simulink model "righttrajectoryagent"  (Simulink 6.2)
settings: Solver=ode45  SolverMode=SingleTasking  StartTime=0.0  StopTime=10.0  RelTol=1e-3  AbsTol=1e-6
settings Model: Creator=The MathWorks Inc.  LastModifiedBy=suarezjl  ExtModeTrigMode=oneshot  ExtModeArmWhenConnect=off  ExtModeAutoUpdateStatusClock=off
settings DataIOCC: LimitDataPoints=off  SignalLoggingName=logsOut
settings OptimizationCC: BooleanDataType=off  InlineInvariantSignals=on
settings DebuggingCC: CheckExecutionContextPreStartOutputMsg=on  CheckExecutionContextRuntimeOutputMsg=on  IntegerOverflowMsg=none
settings HardwareCC: TargetUnknown=on
settings ModelReferenceCC: UpdateModelReferenceTargets=IfOutOfDate

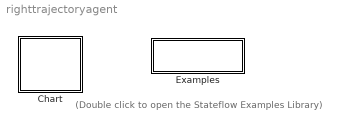
== system righttrajectoryagent ==
  note: (Double click to open the
      | Stateflow Examples Library)
  Chart : Stateflow chart
  Examples : Subsystem
      settings: OpenFcn=sf('Private','sf_examples')
      mask Display: disp('Examples')

== system righttrajectoryagent/Examples ==

== stateflow chart Chart ==
  state InitializeFunctions
    Popeye\RightReachDemo\RightTrajectoryAgent\LoadHomePosition.Initialize()
    Popeye\RightReachDemo\RightTrajectoryAgent\PlayCurrentTraj.Initialize()
    Popeye\RightReachDemo\RightTrajectoryAgent\LoadHomePosition.Write2VS()
  state CopyCurrentLocation
    Popeye\RightReachDemo\RightTrajectoryAgent\CopyGoalPosition.CopyRowVector()
    Popeye\RightReachDemo\RightTrajectoryAgent\CopyCurrentPosition.CopyCurrentVector()
  state GenerateCurrentTrajectory
    Popeye\RightReachDemo\RightTrajectoryAgent\GenerateCurrentTraj.GenerateTrajectory()
  state PlayCurrentTrajectory
    Popeye\RightReachDemo\RightTrajectoryAgent\PlayCurrentTraj.OutputTrajectory()
    Popeye\RightReachDemo\RightTrajectoryAgent\StateMachine.Wait(1000)
  state CopyHomeLocation
    Popeye\RightReachDemo\RightTrajectoryAgent\CopyHomePosition.CopyRowVector()
    Popeye\RightReachDemo\RightTrajectoryAgent\CopyCurrentPosition.CopyCurrentVector()
  state PlayHomeTrajectory
    Popeye\RightReachDemo\RightTrajectoryAgent\PlayCurrentTraj.OutputTrajectory()
  state GenerateHomeTrajectory
    Popeye\RightReachDemo\RightTrajectoryAgent\GenerateCurrentTraj.GenerateTrajectory()
  state Check that object is seen
    Popeye\RightReachDemo\RightTrajectoryAgent\GenerateCurrentTraj.CheckForObject()
  (default) -> InitializeFunctions : Start
  InitializeFunctions -> Check that object is seen : Always
  CopyCurrentLocation -> GenerateCurrentTrajectory : Always
  GenerateCurrentTrajectory -> PlayCurrentTrajectory : Always
  PlayHomeTrajectory -> CopyCurrentLocation : Signal="Next"
  PlayCurrentTrajectory -> CopyHomeLocation : Always
  GenerateHomeTrajectory -> PlayHomeTrajectory : Always
  CopyHomeLocation -> GenerateHomeTrajectory : Always
  Check that object is seen -> CopyCurrentLocation : Signal ="Next"
